simulink model "horno_limitacion_por_rampa"  (R2015a)
settings: Solver=ode45  StartTime=0.0  StopTime=8000  RelTol=1e-3
libraries: simulink x2
settings Model: Creator=m4v  LastModifiedBy=m4v

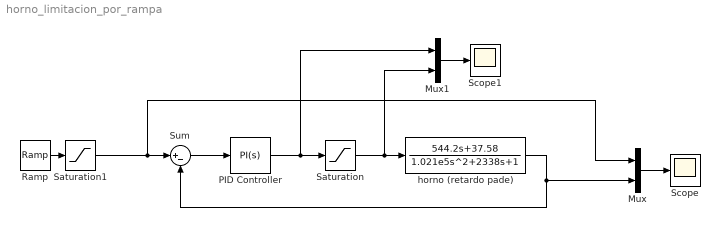
== system horno_limitacion_por_rampa ==
  Mux : Mux  Inputs=2
  Mux1 : Mux  Inputs=2
  PID Controller : simulink/Continuous/PID Controller  Controller=PI  TimeDomain=Continuous-time  SampleTime=-1  IntegratorMethod=Forward Euler  FilterMethod=Forward Euler  Form=Parallel  UseFilter=on  ControllerParametersSource=internal  P=3.5  I=0.0012  D=0  N=100  InitialConditionSource=internal  InitialConditionForIntegrator=0  InitialConditionForFilter=0  ExternalReset=none  LimitOutput=off  UpperSaturationLimit=100  LowerSaturationLimit=0  LinearizeAsGain=on  AntiWindupMode=clamping  Kb=1  TrackingMode=off  Kt=1  PParamMin=[]  PParamMax=[]  IParamMin=[]  IParamMax=[]  DParamMin=[]  DParamMax=[]  NParamMin=[]  NParamMax=[]  KbParamMin=[]  KbParamMax=[]  KtParamMin=[]  KtParamMax=[]  POutMin=[]  POutMax=[]  IOutMin=[]  IOutMax=[]  DOutMin=[]  DOutMax=[]  NOutMin=[]  NOutMax=[]  KbOutMin=[]  KbOutMax=[]  KtOutMin=[]  KtOutMax=[]  IntegratorOutMin=[]  IntegratorOutMax=[]  FilterOutMin=[]  FilterOutMax=[]  SumOutMin=[]  SumOutMax=[]  SumI1OutMin=[]  SumI1OutMax=[]  SumI2OutMin=[]  SumI2OutMax=[]  SumI3OutMin=[]  SumI3OutMax=[]  SumDOutMin=[]  SumDOutMax=[]  SaturationOutMin=[]  SaturationOutMax=[]  IntegratorContinuousStateAttributes=''  IntegratorStateMustResolveToSignalObject=off  IntegratorRTWStateStorageClass=Auto  FilterContinuousStateAttributes=''  FilterStateMustResolveToSignalObject=off  FilterRTWStateStorageClass=Auto  DifferentiatorICPrevScaledInput=0  DifferentiatorOutMin=[]  DifferentiatorOutMax=[]
  Ramp : simulink/Sources/Ramp  slope=0.8  start=0  X0=0
  Saturation : Saturate  UpperLimit=100  LowerLimit=0  ZeroCross=off
  Saturation1 : Saturate  UpperLimit=800  LowerLimit=0
  Scope : Scope
      settings: TimeRange=8000  YMin=0  YMax=900  SampleInput=on  SampleTime=1
  Scope1 : Scope
      settings: TimeRange=8000  YMin=0  YMax=80
  Sum : Sum  Inputs=|+-
  horno (retardo pade) : TransferFcn  Numerator=[544.2 37.58]  Denominator=[1.021e5 2338 1]
  wires:
  Sum/1 -> PID Controller/1
  Mux/1 -> Scope/1
  Mux1/1 -> Scope1/1
  Ramp/1 -> Saturation1/1
  Saturation1/1 -> Mux/1, Sum/1
  PID Controller/1 -> Mux1/1, Saturation/1
  Saturation/1 -> Mux1/2, horno (retardo pade)/1
  horno (retardo pade)/1 -> Mux/2, Sum/2
